simulink model "AttitudePlayground"  (R2024b)
settings: Solver=FixedStepAuto  StartTime=0.0  StopTime=inf  FixedStep=delta_t  RelTol=1e-3  EnableMultiTasking=on
values from neighbouring files (symbols this model uses):
  A = [eye(3), delta_t * eye(3) ... (first row only)    [AttitudePlayground_Vars.m]    (also in ParameterIdentification.m = [0 1)
  A_ESO = [1-l1_ESO, delta_t-l1_ESO*delta_t ... (first row only)    [AttitudePlayground_Vars.m]
  A_kalman = [1 delta_t ... (first row only)    [AttitudePlayground_Vars.m]    (also in ControlSystem_Vars.m)
  acc_sigma = 0.2 * calc_sigma(acc_pp)    [AttitudePlayground_Vars.m]    (also in ControlSystem_Vars.m)
  alpha_comp_pitch = calc_alpha(0.1, delta_t)    [AttitudePlayground_Vars.m]
  alpha_comp_roll = calc_alpha(0.1, delta_t)    [AttitudePlayground_Vars.m]
  alpha_comp_yaw = calc_alpha(1, delta_t)    [AttitudePlayground_Vars.m]
  B = zeros(6,3)    [AttitudePlayground_Vars.m]    (also in ParameterIdentification.m = [0)
  b_ESO = [b0_ESO*delta_t - l1_ESO*b0_ESO*delta_t ... (first row only)    [AttitudePlayground_Vars.m]
  bias_0 = [0, 0, 0]    [AttitudePlayground_Vars.m]
  bias_sigma = 0.000000001    (= 1e-09)    [AttitudePlayground_Vars.m]
  C = eye(6)    [AttitudePlayground_Vars.m]    (also in ParameterIdentification.m = [1 0])
  C_kalman = eye(2)    [AttitudePlayground_Vars.m]    (also in ControlSystem_Vars.m)
  delta_t = 0.01    [AttitudePlayground_Vars.m]    (also in ControlSystem_Vars.m; ParameterIdentification.m = t2 - t1)
  gyro_sigma = 1*((pi/180) * (0.07))    (= 0.0012217304764)    [AttitudePlayground_Vars.m]    (also in ControlSystem_Vars.m)
  gyro_sigma_3d = [1*gyro_sigma, 1*gyro_sigma, gyro_sigma]    [AttitudePlayground_Vars.m]    (also in ControlSystem_Vars.m)
  k_i_mahony = 0.0057    [AttitudePlayground_Vars.m]
  k_p_mahony = 0.42    [AttitudePlayground_Vars.m]
  l = [l1_ESO, l2_ESO]'    [AttitudePlayground_Vars.m]
  mag_sigma = 0.8 * calc_sigma(mag_pp)    [AttitudePlayground_Vars.m]
  P_0 = eye(4)    [AttitudePlayground_Vars.m]    (also in ControlSystem_Vars.m)
  P_0_gb = eye(7)    [AttitudePlayground_Vars.m]
  q_init = [cos(initial_yaw/2), 0, 0, sin(initial_yaw/2)]    [AttitudePlayground_Vars.m]
  q_sigma = 0.001    [AttitudePlayground_Vars.m]    (also in ControlSystem_Vars.m)
  R = 1.8 * diag([0.001396263^2, 0.0016580628^2, 0.05^2, ((pi/180) *              (0.05))^2, ((pi/180) * (0.07))^2, ((pi/180) * (0.07))^2])    [AttitudePlayground_Vars.m]    (also in ControlSystem_Vars.m = 0.015625)
  R_kalman = diag([(calc_sigma(0.8))^2, (0.07)^2])    [AttitudePlayground_Vars.m]    (also in ControlSystem_Vars.m)
  r_qekf = 1/sqrt(cos(magnetic_dip_angle_theta)^2 +      sin(magnetic_dip_angle_theta)^2)  * transpose([cos(magnetic_dip_angle_theta),0, sin(magnetic_dip_angle_theta)])    [AttitudePlayground_Vars.m]
  step_time = 10    [AttitudePlayground_Vars.m]
  tau_pitch_comp = 0.5    [AttitudePlayground_Vars.m]
  tau_roll_comp = 0.5    [AttitudePlayground_Vars.m]
  tau_yaw_comp = 3    [AttitudePlayground_Vars.m]
  Ts = delta_t    (= 0.01)    [AttitudePlayground_Vars.m]
  Ts2 = delta_t/2    (= 0.005)    [AttitudePlayground_Vars.m]
  Ts_IMU = delta_t    (= 0.01)    [AttitudePlayground_Vars.m]
  voltage_divider_Vout_max = 1.728    [AttitudePlayground_Vars.m]
undefined symbols (not defined in the file or in its folder): DiscIntNeverNeededParam, Discrete, Newton, Raphson, Time
libraries: simulink_extras x26, dspsigops x5, bbblueActuatorLib x4, ctrlSharedLib x2, matrix_library x2, dspmathops x2, dspstat3 x1, bbblueSensorLib x1, simulink x1, dspfdesign x1, bbblueBasicLib x1, vrlib x1
(part 3 of 3)

== matlab function AttitudePlayground/Quarternion EKF + Amfitrack (Yaw Only)/Update ==
  data: accel input; q_meas input; q_t output; quat_in input; acc_sigma input; q_sigma input; P_t output; P_t_dash input; prev_yaw_mp input; prev_cul_yaw_mp input; yaw_mp output; yaw_cul_mp output
function [q_t, P_t, yaw_mp, yaw_cul_mp]   = Update(accel, q_meas, quat_in, acc_sigma, q_sigma, P_t_dash, prev_yaw_mp, prev_cul_yaw_mp)

%% Unbox function inputs
q0 = quat_in(1);
q1 = quat_in(2);
q2 = quat_in(3);
q3 = quat_in(4);

q_t_dash = [q0; q1; q2; q3];

yaw_meas_prev = prev_yaw_mp(1);
yaw_meas_cul_prev = prev_cul_yaw_mp(1);
yaw_pred_prev = prev_yaw_mp(2);
yaw_pred_cul_prev = prev_cul_yaw_mp(2);

yaw_meas = atan2((2 * (q_meas(1)*q_meas(4) + q_meas(2)*q_meas(3))),(1 - 2*(q_meas(3)^2 + q_meas(4)^2)));
yaw_pred = atan2((2 * (q0*q3 + q1*q2)),(1 - 2*(q2^2 + q3^2)));

%% Accumulate measured & predicted Yaw Angles
% Determine Change in measured and predicted Yaw angle
delta_yaw_meas = yaw_meas - yaw_meas_prev;
delta_yaw_pred = yaw_pred - yaw_pred_prev;

if delta_yaw_meas > pi
    delta_yaw_meas = delta_yaw_meas - 2*pi;
elseif delta_yaw_meas < -pi
    delta_yaw_meas = delta_yaw_meas + 2*pi;
end

yaw_meas_cul = yaw_meas_cul_prev + delta_yaw_meas;

if delta_yaw_pred > pi
    delta_yaw_pred = delta_yaw_pred - 2*pi;
elseif delta_yaw_pred < -pi
    delta_yaw_pred = delta_yaw_pred + 2*pi;
end

yaw_pred_cul = yaw_pred_cul_prev + delta_yaw_pred;

% Send them to the delay blocks for use in next update step
yaw_mp = [yaw_meas,yaw_pred];
yaw_cul_mp = [yaw_meas_cul, yaw_pred_cul];


%% Update State Estimation

% Construct measurement vector using accumulated yaw angles
z_t = [accel(1);
       accel(2);
       accel(3);
       yaw_meas_cul;
       ];

gx = 0;
gy = 0;
gz = 1;

R = [acc_sigma^2 * eye(3) zeros(3,1);
    zeros(1,3)     q_sigma^2 * eye(1)];

% Measurement Model
h = [
    2*(gx * (1/2 - q2^2 - q3^2) + gy * (q0*q3 + q1*q2) + gz * (q1*q3 - q0*q2));
    2*(gx * (q1*q2 - q0*q3) + gy * (1/2 - q1^2 - q3^2) + gz * (q0*q1 + q2*q3));
    2*(gx * (q0*q2 + q1*q3) + gy * (q2*q3 - q0*q1) + gz * (1/2 - q1^2 - q2^2));
                                    yaw_pred_cul                           ;
                                    
];

% Jacobian of Measurement Model
H = 2 * [
    gx*q0 + gy*q3 - gz*q2,  gx*q1 + gy*q2 + gz*q3, -gx*q2 + gy*q1 - gz*q0, -gx*q3 + gy*q0 + gz*q1;
   -gx*q3 + gy*q0 + gz*q1,  gx*q2 - gy*q1 + gz*q0,  gx*q1 + gy*q2 + gz*q3, -gx*q0 - gy*q3 + gz*q2;
    gx*q2 - gy*q1 + gz*q0,  gx*q3 - gy*q0 - gz*q1,  gx*q0 + gy*q3 - gz*q2,  gx*q1 + gy*q2 + gz*q3;
                                            
    0.5*[-(2*q3*(2*q2^2 + 2*q3^2 - 1))/((2*q2^2 + 2*q3^2 - 1)^2 + (2*q0*q3 + 2*q1*q2)^2), -(2*q2*(2*q2^2 + 2*q3^2 - 1))/((2*q2^2 + 2*q3^2 - 1)^2 + (2*q0*q3 + 2*q1*q2)^2), -(((2*q1)/(2*q2^2 + 2*q3^2 - 1) - (4*q2*(2*q0*q3 + 2*q1*q2))/(2*q2^2 + 2*q3^2 - 1)^2)*(2*q2^2 + 2*q3^2 - 1)^2)/((2*q2^2 + 2*q3^2 - 1)^2 + (2*q0*q3 + 2*q1*q2)^2), -(((2*q0)/(2*q2^2 + 2*q3^2 - 1) - (4*q3*(2*q0*q3 + 2*q1*q2))/(2*q2^2 + 2*q3^2 - 1)^2)*(2*q2^2 + 2*q3^2 - 1)^2)/((2*q2^2 + 2*q3^2 - 1)^2 + (2*q0*q3 + 2*q1*q2)^2)]
];

v_t = z_t - h;

S_t = H * P_t_dash * transpose(H) + R;
K_t = P_t_dash * transpose(H) * inv(S_t);

q_t = quatnormalize(transpose(q_t_dash + K_t*v_t));

P_t = (eye(4) - K_t*H) * P_t_dash;

== matlab function AttitudePlayground/Quarternion EKF + Amfitrack (Yaw Only)/normalize_g_b ==
  data: v input; v_norm output
function v_norm = normalize_vec(v)

v_norm = v / norm(v);

== matlab function AttitudePlayground/Quarternion EKF + Amfitrack (Yaw Only)1/MATLAB Function ==
  data: quat_in input; euler output
function euler = to_euler(quat_in)

q0 = quat_in(1);
q1 = quat_in(2);
q2 = quat_in(3);
q3 = quat_in(4);

roll = atan((2 * (q0*q1 + q2*q3))/(1 - 2*(q1^2 + q2^2)));
pitch = asin(2 * (q0*q2 - q1*q3));
yaw = atan2((2 * (q0*q3 + q1*q2)),(1 - 2*(q2^2 + q3^2)));

euler = [roll; pitch; yaw];

== matlab function AttitudePlayground/Quarternion EKF + Amfitrack (Yaw Only)1/Predict ==
  data: quat_in input; q_t_dash output; omega input; delta_t input; P_t_dash output; P_t_ input; gyro_sigma input
function [q_t_dash, P_t_dash] = Predict(quat_in, omega, delta_t, P_t_, gyro_sigma)

q0 = quat_in(1);
q1 = quat_in(2);
q2 = quat_in(3);
q3 = quat_in(4);

omega_x = omega(1);
omega_y = omega(2);
omega_z = omega(3);

R_gyro = [gyro_sigma(1)^2 0 0;
          0 gyro_sigma(2)^2 0;
          0 0 gyro_sigma(3)^2;];

q0_out = q0 + delta_t/2 * (-omega_x * q1 - omega_y * q2 - omega_z * q3);
q1_out = q1 + delta_t/2 * ( omega_x * q0 - omega_y * q3 + omega_z * q2);
q2_out = q2 + delta_t/2 * ( omega_x * q3 + omega_y * q0 - omega_z * q1);
q3_out = q3 + delta_t/2 * (-omega_x * q2 + omega_y * q1 + omega_z * q0);

q_t_dash = quatnormalize([q0_out, q1_out, q2_out, q3_out]);

dt2 = delta_t/2;

F = [1  -dt2*omega_x -dt2*omega_y -dt2*omega_z;
    dt2*omega_x    1  dt2*omega_z  dt2*omega_y;
    dt2*omega_y   -dt2*omega_z   1 dt2*omega_x;
    dt2*omega_z    dt2*omega_y -dt2*omega_x  1;
    ];


W = dt2 * [-q1 -q2 -q3;
            q0 -q3  q2;
            q3  q0 -q1;
            -q2 q1  q0]; 

Q_t =  W* R_gyro * W';

P_t_dash = F * P_t_ * F' + Q_t;

== matlab function AttitudePlayground/Quarternion EKF + Amfitrack (Yaw Only)1/Update ==
  data: accel input; q_meas input; q_t output; quat_in input; acc_sigma input; q_sigma input; P_t output; P_t_dash input; prev_yaw_mp input; prev_cul_yaw_mp input; yaw_mp output; yaw_cul_mp output
function [q_t, P_t, yaw_mp, yaw_cul_mp]   = Update(accel, q_meas, quat_in, acc_sigma, q_sigma, P_t_dash, prev_yaw_mp, prev_cul_yaw_mp)

%% Unbox function inputs
q0 = quat_in(1);
q1 = quat_in(2);
q2 = quat_in(3);
q3 = quat_in(4);

q_t_dash = [q0; q1; q2; q3];

yaw_meas_prev = prev_yaw_mp(1);
yaw_meas_cul_prev = prev_cul_yaw_mp(1);
yaw_pred_prev = prev_yaw_mp(2);
yaw_pred_cul_prev = prev_cul_yaw_mp(2);

yaw_meas = atan2((2 * (q_meas(1)*q_meas(4) + q_meas(2)*q_meas(3))),(1 - 2*(q_meas(3)^2 + q_meas(4)^2)));
yaw_pred = atan2((2 * (q0*q3 + q1*q2)),(1 - 2*(q2^2 + q3^2)));

%% Accumulate measured & predicted Yaw Angles
% Determine Change in measured and predicted Yaw angle
delta_yaw_meas = yaw_meas - yaw_meas_prev;
delta_yaw_pred = yaw_pred - yaw_pred_prev;

if delta_yaw_meas > pi
    delta_yaw_meas = delta_yaw_meas - 2*pi;
elseif delta_yaw_meas < -pi
    delta_yaw_meas = delta_yaw_meas + 2*pi;
end

yaw_meas_cul = yaw_meas_cul_prev + delta_yaw_meas;

if delta_yaw_pred > pi
    delta_yaw_pred = delta_yaw_pred - 2*pi;
elseif delta_yaw_pred < -pi
    delta_yaw_pred = delta_yaw_pred + 2*pi;
end

yaw_pred_cul = yaw_pred_cul_prev + delta_yaw_pred;

% Send them to the delay blocks for use in next update step
yaw_mp = [yaw_meas,yaw_pred];
yaw_cul_mp = [yaw_meas_cul, yaw_pred_cul];

%% Update prediction quaternion to represent accumulated yaw
roll = atan((2 * (q0*q1 + q2*q3))/(1 - 2*(q1^2 + q2^2)));
pitch = asin(2 * (q0*q2 - q1*q3));
yaw = yaw_pred_cul;

q_pred_updated = eul2quat([yaw pitch roll]);

q0 = q_pred_updated(1);
q1 = q_pred_updated(2);
q2 = q_pred_updated(3);
q3 = q_pred_updated(4);

%% Update State Estimation

% Construct measurement vector using accumulated yaw angles
z_t = [accel(1);
       accel(2);
       accel(3);
       cos(yaw_meas_cul/2);
       0;
       0;
       sin(yaw_meas_cul/2)
         ];

gx = 0;
gy = 0;
gz = 1;

R = [acc_sigma^2 * eye(3) zeros(3,4);
    zeros(4,3)     q_sigma^2 * eye(4)];

% Measurement Model
h = [
    2*(gx * (1/2 - q2^2 - q3^2) + gy * (q0*q3 + q1*q2) + gz * (q1*q3 - q0*q2));
    2*(gx * (q1*q2 - q0*q3) + gy * (1/2 - q1^2 - q3^2) + gz * (q0*q1 + q2*q3));
    2*(gx * (q0*q2 + q1*q3) + gy * (q2*q3 - q0*q1) + gz * (1/2 - q1^2 - q2^2));
                                    cos(yaw_pred_cul/2)                           ;
                                    0                                         ;
                                    0                                         ;
                                    sin(yaw_pred_cul/2)                           ;
];

% Jacobian of Measurement Model
H = 2 * [
    gx*q0 + gy*q3 - gz*q2,  gx*q1 + gy*q2 + gz*q3, -gx*q2 + gy*q1 - gz*q0, -gx*q3 + gy*q0 + gz*q1;
   -gx*q3 + gy*q0 + gz*q1,  gx*q2 - gy*q1 + gz*q0,  gx*q1 + gy*q2 + gz*q3, -gx*q0 - gy*q3 + gz*q2;
    gx*q2 - gy*q1 + gz*q0,  gx*q3 - gy*q0 - gz*q1,  gx*q0 + gy*q3 - gz*q2,  gx*q1 + gy*q2 + gz*q3;
                                            
    0.5*[(q3*sin(atan2((2*q0*q3 + 2*q1*q2), - 2*q2^2 - 2*q3^2 + 1)/2)*(2*q2^2 + 2*q3^2 - 1))/((2*q2^2 + 2*q3^2 - 1)^2 + (2*q0*q3 + 2*q1*q2)^2), (q2*sin(atan2((2*q0*q3 + 2*q1*q2), - 2*q2^2 - 2*q3^2 + 1)/2)*(2*q2^2 + 2*q3^2 - 1))/((2*q2^2 + 2*q3^2 - 1)^2 + (2*q0*q3 + 2*q1*q2)^2), (sin(atan2((2*q0*q3 + 2*q1*q2), - 2*q2^2 - 2*q3^2 + 1)/2)*((2*q1)/(2*q2^2 + 2*q3^2 - 1) - (4*q2*(2*q0*q3 + 2*q1*q2))/(2*q2^2 + 2*q3^2 - 1)^2)*(2*q2^2 + 2*q3^2 - 1)^2)/(2*((2*q2^2 + 2*q3^2 - 1)^2 + (2*q0*q3 + 2*q1*q2)^2)), (sin(atan2((2*q0*q3 + 2*q1*q2), - 2*q2^2 - 2*q3^2 + 1)/2)*((2*q0)/(2*q2^2 + 2*q3^2 - 1) - (4*q3*(2*q0*q3 + 2*q1*q2))/(2*q2^2 + 2*q3^2 - 1)^2)*(2*q2^2 + 2*q3^2 - 1)^2)/(2*((2*q2^2 + 2*q3^2 - 1)^2 + (2*q0*q3 + 2*q1*q2)^2)); 
    0, 0, 0, 0; 
    0, 0, 0, 0; 
    -(q3*cos(atan2((2*q0*q3 + 2*q1*q2), - 2*q2^2 - 2*q3^2 + 1)/2)*(2*q2^2 + 2*q3^2 - 1))/((2*q2^2 + 2*q3^2 - 1)^2 + (2*q0*q3 + 2*q1*q2)^2), -(q2*cos(atan2((2*q0*q3 + 2*q1*q2), - 2*q2^2 - 2*q3^2 + 1)/2)*(2*q2^2 + 2*q3^2 - 1))/((2*q2^2 + 2*q3^2 - 1)^2 + (2*q0*q3 + 2*q1*q2)^2), -(cos(atan2((2*q0*q3 + 2*q1*q2), - 2*q2^2 - 2*q3^2 + 1)/2)*((2*q1)/(2*q2^2 + 2*q3^2 - 1) - (4*q2*(2*q0*q3 + 2*q1*q2))/(2*q2^2 + 2*q3^2 - 1)^2)*(2*q2^2 + 2*q3^2 - 1)^2)/(2*((2*q2^2 + 2*q3^2 - 1)^2 + (2*q0*q3 + 2*q1*q2)^2)), -(cos(atan2((2*q0*q3 + 2*q1*q2), - 2*q2^2 - 2*q3^2 + 1)/2)*((2*q0)/(2*q2^2 + 2*q3^2 - 1) - (4*q3*(2*q0*q3 + 2*q1*q2))/(2*q2^2 + 2*q3^2 - 1)^2)*(2*q2^2 + 2*q3^2 - 1)^2)/(2*((2*q2^2 + 2*q3^2 - 1)^2 + (2*q0*q3 + 2*q1*q2)^2))]
];

v_t = z_t - h;

S_t = H * P_t_dash * transpose(H) + R;
K_t = P_t_dash * transpose(H) * inv(S_t);

q_t = quatnormalize(transpose(q_t_dash + K_t*v_t));

P_t = (eye(4) - K_t*H) * P_t_dash;

== matlab function AttitudePlayground/Quarternion EKF + Amfitrack (Yaw Only)1/normalize_g_b ==
  data: v input; v_norm output
function v_norm = normalize_vec(v)

v_norm = v / norm(v);

== matlab function AttitudePlayground/Quarternion EKF + Amfitrack (Yaw Only)/Initialize QEKF_AOY ==
  data: quat_meas input; q_init output
function q_init = calc_init_q(quat_meas)

q0 = quat_meas(1);
q1 = quat_meas(2);
q2 = quat_meas(3);
q3 = quat_meas(4);


yaw_init_rad = atan2((2 * (q0*q3 + q1*q2)),(1 - 2*(q2^2 + q3^2)));
q_init = [cos(yaw_init_rad/2), 0, 0, sin(yaw_init_rad/2)];

== matlab function AttitudePlayground/Angles from Accel + Mag/MATLAB Function2 ==
  data: roll input; pitch input; m_x input; yaw output; m_y input; m_z input
function yaw = calc_yaw(roll, pitch, m_x, m_y, m_z)
    % Adjust for roll
    m_x2 = m_x * cos(pitch) + m_z * sin(pitch);
    m_y2 = m_x * sin(roll) * sin(pitch) + m_y * cos(roll) - m_z * sin(roll) * cos(pitch);
    % Calculate yaw
    yaw = atan2(-m_y2, m_x2);



%function yaw = calc_yaw(a_x, pitch, roll, m_x, m_y, m_z)

%m_y2 = m_z * sin(roll) - m_y * cos(roll);
%m_z2 = m_y * sin(roll) - m_z * cos(roll);
%m_x2 = m_x * cos(pitch) + m_z2 * sin(pitch);
%yaw = atan(m_y2/m_x2);

%yaw = atan(-a_x / (m_x*cos(roll)) + ...
%            m_y * sin(roll) * sin(pitch) + ...
%            m_z * cos(roll)  *sin(pitch));

== matlab function AttitudePlayground/Leightweight-Kalman/Initialize KF ==
  data: quat_meas input; q_init output
function q_init = calc_init_q(quat_meas)

q0 = quat_meas(1);
q1 = quat_meas(2);
q2 = quat_meas(3);
q3 = quat_meas(4);


yaw_init_rad = atan2((2 * (q0*q3 + q1*q2)),(1 - 2*(q2^2 + q3^2)));
q_init = [cos(yaw_init_rad/2), 0, 0, sin(yaw_init_rad/2)];

== matlab function AttitudePlayground/Leightweight-Kalman/MATLAB Function1 ==
  data: quat_in input; euler output
function euler = to_euler(quat_in)

q0 = quat_in(1);
q1 = quat_in(2);
q2 = quat_in(3);
q3 = quat_in(4);

roll = atan((2 * (q0*q1 + q2*q3))/(1 - 2*(q1^2 + q2^2)));
pitch = asin(2 * (q0*q2 - q1*q3));
yaw = atan2((2 * (q0*q3 + q1*q2)),(1 - 2*(q2^2 + q3^2)));

euler = [roll; pitch; yaw];

== matlab function AttitudePlayground/Leightweight-Kalman/MATLAB Function2 ==
  data: quat_in input; euler output
function euler = to_euler(quat_in)

q0 = quat_in(1);
q1 = quat_in(2);
q2 = quat_in(3);
q3 = quat_in(4);

roll = atan((2 * (q0*q1 + q2*q3))/(1 - 2*(q1^2 + q2^2)));
pitch = asin(2 * (q0*q2 - q1*q3));
yaw = atan2((2 * (q0*q3 + q1*q2)),(1 - 2*(q2^2 + q3^2)));

euler = [roll; pitch; yaw];

== matlab function AttitudePlayground/Mahony+Bias-Estimator/normalize_g_b ==
  data: g_b input; g_b_norm output
function g_b_norm = fcn(g_b)

g_b_norm = g_b / norm(g_b);

== matlab function AttitudePlayground/Mahony+Bias-Estimator/MATLAB Function1 ==
  data: euler output; omega input; delta_t input; quat_mem input; quaternion_tplus output
function [euler, quaternion_tplus] = fcn(omega, delta_t, quat_mem)

q0 = quat_mem(1);
q1 = quat_mem(2);
q2 = quat_mem(3);
q3 = quat_mem(4);

omega_x = omega(1);
omega_y = omega(2);
omega_z = omega(3);

q0_tp = q0 + delta_t/2 * (-omega_x * q1 - omega_y * q2 - omega_z * q3);
q1_tp = q1 + delta_t/2 * ( omega_x * q0 + omega_z * q2 - omega_y * q3);
q2_tp = q2 + delta_t/2 * ( omega_y * q0 - omega_z * q1 + omega_z * q3);
q3_tp = q3 + delta_t/2 * ( omega_z * q0 + omega_y * q1 - omega_x * q2);

quaternion_tplus = [q0_tp, q1_tp, q2_tp, q3_tp];

roll = atan((2 * (q0_tp*q1_tp + q2_tp*q3_tp))/(1 - 2*(q1_tp^2 + q2_tp^2)));
pitch = asin(2 * (q0_tp*q2_tp - q1_tp*q3_tp));
yaw = atan2((2 * (q0_tp*q3_tp + q1_tp*q2_tp)),(1 - 2*(q2_tp^2 + q3_tp^2)));

euler = [roll; pitch; yaw];

== matlab function AttitudePlayground/Mahony+Bias-Estimator/MATLAB Function2 ==
  data: q input; v_b output
function v_b = fcn(q)

q0 = q(1);
q1 = q(2);
q2 = q(3);
q3 = q(4);
v_b = [2*(q1*q3 - q0*q2);
       2*(q0*q1 + q2*q3);
       1 - 2*(q1^2 + q2^2)];

== matlab function AttitudePlayground/Quarternion EKF/Update ==
  data: accel input; mag input; q_t output; quat_in input; r input; acc_sigma input; mag_sigma input; P_t output; P_t_dash input
function [q_t, P_t]   = Update(accel, mag, quat_in, r, acc_sigma, mag_sigma, P_t_dash)

q0 = quat_in(1);
q1 = quat_in(2);
q2 = quat_in(3);
q3 = quat_in(4);

q_t_dash = [q0; q1; q2; q3];

z_t = [accel(1);
       accel(2);
       accel(3);
         mag(1);
         mag(2);
         mag(3);];

rx = r(1);
ry = r(2);
rz = r(3);
gx = 0;
gy = 0;
gz = 1;

R = [acc_sigma^2 * eye(3) zeros(3);
    zeros(3)     mag_sigma^2 * eye(3)];


h = 2 * [
    gx * (1/2 - q2^2 - q3^2) + gy * (q0*q3 + q1*q2) + gz * (q1*q3 - q0*q2);
    gx * (q1*q2 - q0*q3) + gy * (1/2 - q1^2 - q3^2) + gz * (q0*q1 + q2*q3);
    gx * (q0*q2 + q1*q3) + gy * (q2*q3 - q0*q1) + gz * (1/2 - q1^2 - q2^2);
    rx * (1/2 - q2^2 - q3^2) + ry * (q0*q3 + q1*q2) + rz * (q1*q3 - q0*q2);
    rx * (q1*q2 - q0*q3) + ry * (1/2 - q1^2 - q3^2) + rz * (q0*q1 + q2*q3);
    rx * (q0*q2 + q1*q3) + ry * (q2*q3 - q0*q1) + rz * (1/2 - q1^2 - q2^2)
];

H = 2 * [
    gx*q0 + gy*q3 - gz*q2,  gx*q1 + gy*q2 + gz*q3, -gx*q2 + gy*q1 - gz*q0, -gx*q3 + gy*q0 + gz*q1;
   -gx*q3 + gy*q0 + gz*q1,  gx*q2 - gy*q1 + gz*q0,  gx*q1 + gy*q2 + gz*q3, -gx*q0 - gy*q3 + gz*q2;
    gx*q2 - gy*q1 + gz*q0,  gx*q3 - gy*q0 - gz*q1,  gx*q0 + gy*q3 - gz*q2,  gx*q1 + gy*q2 + gz*q3;
    rx*q0 + ry*q3 - rz*q2,  rx*q1 + ry*q2 + rz*q3, -rx*q2 + ry*q1 - rz*q0, -rx*q3 + ry*q0 + rz*q1;
   -rx*q3 + ry*q0 + rz*q1,  rx*q2 - ry*q1 + rz*q0,  rx*q1 + ry*q2 + rz*q3, -rx*q0 - ry*q3 + rz*q2;
    rx*q2 - ry*q1 + rz*q0,  rx*q3 - ry*q0 - rz*q1,  rx*q0 + ry*q3 - rz*q2,  rx*q1 + ry*q2 + rz*q3
];

v_t = z_t - h;

S_t = H * P_t_dash * transpose(H) + R;
K_t = P_t_dash * transpose(H) * inv(S_t);

q_t = quatnormalize(transpose(q_t_dash + K_t*v_t));

P_t = (eye(4) - K_t*H) * P_t_dash;

== matlab function AttitudePlayground/Quarternion EKF/Predict ==
  data: quat_in input; q_t_dash output; omega input; delta_t input; P_t_dash output; P_t_ input; gyro_sigma input
function [q_t_dash, P_t_dash] = Predict(quat_in, omega, delta_t, P_t_, gyro_sigma)

q0 = quat_in(1);
q1 = quat_in(2);
q2 = quat_in(3);
q3 = quat_in(4);

omega_x = omega(1);
omega_y = omega(2);
omega_z = omega(3);

q0_out = q0 + delta_t/2 * (-omega_x * q1 - omega_y * q2 - omega_z * q3);
q1_out = q1 + delta_t/2 * ( omega_x * q0 - omega_y * q3 + omega_z * q2);
q2_out = q2 + delta_t/2 * ( omega_x * q3 + omega_y * q0 - omega_z * q1);
q3_out = q3 + delta_t/2 * (-omega_x * q2 + omega_y * q1 + omega_z * q0);

q_t_dash = quatnormalize([q0_out, q1_out, q2_out, q3_out]);

dt2 = delta_t/2;

F = [1  -dt2*omega_x -dt2*omega_y -dt2*omega_z;
    dt2*omega_x    1  dt2*omega_z  dt2*omega_y;
    dt2*omega_y   -dt2*omega_z   1 dt2*omega_x;
    dt2*omega_z    dt2*omega_y -dt2*omega_x  1;
    ];


W = dt2 * [-q1 -q2 -q3;
            q0 -q3  q2;
            q3  q0 -q1;
            -q2 q1  q0]; 

Q_t =  gyro_sigma^2 * (W * W');

P_t_dash = F * P_t_ * F' + Q_t;
